simulink model "Fuzzy_PIcontrol"  (Simulink 8.5)
settings: Solver=ode45  StartTime=0.0  StopTime=2500  RelTol=1e-3
libraries: fuzblock x1, simulink x1
settings Model: Creator=YH  LastModifiedBy=YH
settings DataIOCC: SignalLoggingSaveFormat=Dataset
settings OptimizationCC: ExpressionDepthLimit=128
settings DebuggingCC: UnderspecifiedInitializationDetection=Simplified  MergeDetectMultiDrivingBlocksExec=error  FcnCallInpInsideContextMsg=EnableAllAsError  StateNameClashWarn=none
settings GRTTargetCC: CombineOutputUpdateFcns=on  GRTInterface=off

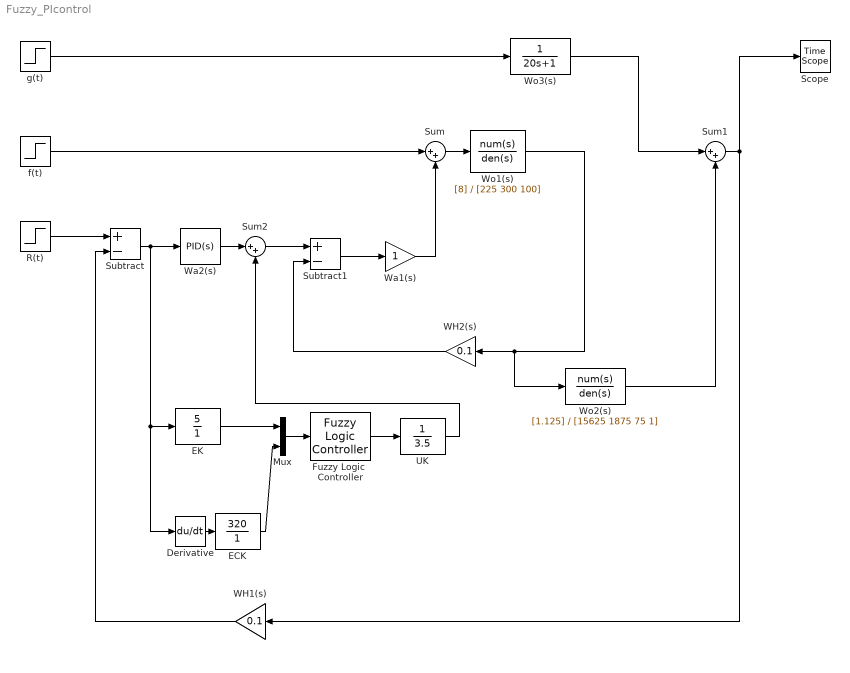
== system Fuzzy_PIcontrol ==
  Derivative : Derivative
  "ECK " : TransferFcn  Numerator=[320]  Denominator=[1]
  EK : TransferFcn  Numerator=[5]  Denominator=[1]
  Fuzzy Logic  Controller : fuzblock/Fuzzy Logic  Controller  RequirementInfo="{}  %GIDa_259873ff_522e_4624_ad10_7ae7b59efd04"  fis=fuzzyController
  Mux : Mux  Inputs=2
  R(t) : Step  SampleTime=0
  Scope : TimeScope
  Subtract : Sum  Inputs=+-
  Subtract1 : Sum  Inputs=+-
  Sum : Sum  Inputs=|++
  Sum1 : Sum  Inputs=|++
  Sum2 : Sum  Inputs=|++
  UK : TransferFcn  Denominator=[3.5]
  WH1(s) : Gain  Gain=0.1
  WH2(s) : Gain  Gain=0.1
  Wa1(s) : Gain
  Wa2(s) : simulink/Continuous/PID Controller  Controller=PID  TimeDomain=Continuous-time  SampleTime=-1  IntegratorMethod=Forward Euler  FilterMethod=Forward Euler  Form=Parallel  UseFilter=on  ControllerParametersSource=internal  P=1  I=1  D=0  N=100  InitialConditionSource=internal  InitialConditionForIntegrator=0  InitialConditionForFilter=0  ExternalReset=none  LimitOutput=off  UpperSaturationLimit=inf  LowerSaturationLimit=-inf  LinearizeAsGain=on  AntiWindupMode=none  Kb=1  TrackingMode=off  Kt=1  PParamMin=[]  PParamMax=[]  IParamMin=[]  IParamMax=[]  DParamMin=[]  DParamMax=[]  NParamMin=[]  NParamMax=[]  KbParamMin=[]  KbParamMax=[]  KtParamMin=[]  KtParamMax=[]  POutMin=[]  POutMax=[]  IOutMin=[]  IOutMax=[]  DOutMin=[]  DOutMax=[]  NOutMin=[]  NOutMax=[]  KbOutMin=[]  KbOutMax=[]  KtOutMin=[]  KtOutMax=[]  IntegratorOutMin=[]  IntegratorOutMax=[]  FilterOutMin=[]  FilterOutMax=[]  SumOutMin=[]  SumOutMax=[]  SumI1OutMin=[]  SumI1OutMax=[]  SumI2OutMin=[]  SumI2OutMax=[]  SumI3OutMin=[]  SumI3OutMax=[]  SumDOutMin=[]  SumDOutMax=[]  SaturationOutMin=[]  SaturationOutMax=[]  IntegratorContinuousStateAttributes=''  IntegratorStateMustResolveToSignalObject=off  IntegratorRTWStateStorageClass=Auto  FilterContinuousStateAttributes=''  FilterStateMustResolveToSignalObject=off  FilterRTWStateStorageClass=Auto  DifferentiatorICPrevScaledInput=0  DifferentiatorOutMin=[]  DifferentiatorOutMax=[]
  Wo1(s) : TransferFcn  Numerator=[8]  Denominator=[225 300 100]
  Wo2(s) : TransferFcn  Numerator=[1.125]  Denominator=[15625 1875 75 1]
  Wo3(s) : TransferFcn  Denominator=[20 1]
  f(t) : Step  Time=900  After=100  SampleTime=0
  g(t) : Step  Time=300  After=10  SampleTime=0
  wires:
  R(t)/1 -> Subtract/1
  WH1(s)/1 -> Subtract/2
  Sum1/1 -> Scope/1, WH1(s)/1
  g(t)/1 -> Wo3(s)/1
  Wo3(s)/1 -> Sum1/1
  Wo1(s)/1 -> Wo2(s)/1, WH2(s)/1
  Wo2(s)/1 -> Sum1/2
  Sum/1 -> Wo1(s)/1
  f(t)/1 -> Sum/1
  Wa1(s)/1 -> Sum/2
  Subtract1/1 -> Wa1(s)/1
  Subtract/1 -> Derivative/1, EK/1, Wa2(s)/1
  WH2(s)/1 -> Subtract1/2
  Wa2(s)/1 -> Sum2/1
  Sum2/1 -> Subtract1/1
  Derivative/1 -> "ECK "/1
  Mux/1 -> Fuzzy Logic  Controller/1
  Fuzzy Logic  Controller/1 -> UK/1
  UK/1 -> Sum2/2
  EK/1 -> Mux/1
  "ECK "/1 -> Mux/2
